simulink model "step_in"  (R2020a)
settings: Solver=ode4  StartTime=0.0  StopTime=10  RelTol=1e-3
settings Model: Creator=18423  LastModifiedBy=18423

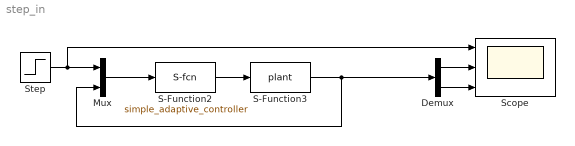
== system step_in ==
  Demux : Demux  Outputs=2
  Mux : Mux  Inputs=2
  S-Function2 : S-Function  FunctionName=simple_adaptive_controller  SFunctionDeploymentMode=off  EnableBusSupport=off
  S-Function3 : S-Function  FunctionName=plant  SFunctionDeploymentMode=off  EnableBusSupport=off
  Scope : Scope  NumInputPorts=3
  Step : Step  After=0.5  SampleTime=0
  wires:
  Step/1 -> Scope/1, Mux/1
  Mux/1 -> S-Function2/1
  S-Function2/1 -> S-Function3/1
  S-Function3/1 -> Demux/1, Mux/2
  Demux/1 -> Scope/2
  Demux/2 -> Scope/3
